simulink model "Bebop_controller_sim"  (R2018a)
settings: Solver=VariableStepAuto  StartTime=0.0  StopTime=25  RelTol=1e-3
values from neighbouring files (symbols this model uses):
  goal = [10 10]    [AnytimeRRT.m]    (also in Plot_sim.m = [rand()*5+20 rand()*-5]; RRTstardy.m = [9 9])
  I = [1 0 0 ... (first row only)    [Bebop_sim_init.m]
  mass = 2    [Bebop_sim_init.m]
  max_rot_Z = (90)*pi/180    (= 1.57079632679)    [Bebop_sim_init.m]
  max_theta_X = (40)*pi/180    (= 0.698131700798)    [Bebop_sim_init.m]
  max_theta_Y = (40)*pi/180    (= 0.698131700798)    [Bebop_sim_init.m]
  max_v_Z = 1.5    [Bebop_sim_init.m]
  start = [0 0]    [AnytimeRRT.m]    (also in Plot_sim.m; RRTstardy.m)
undefined symbols (not defined in the file or in its folder): data
libraries: simulink x6, aerolibactuator x2, shared6dof x1
settings Model: Creator=derek  LastModifiedBy=derek

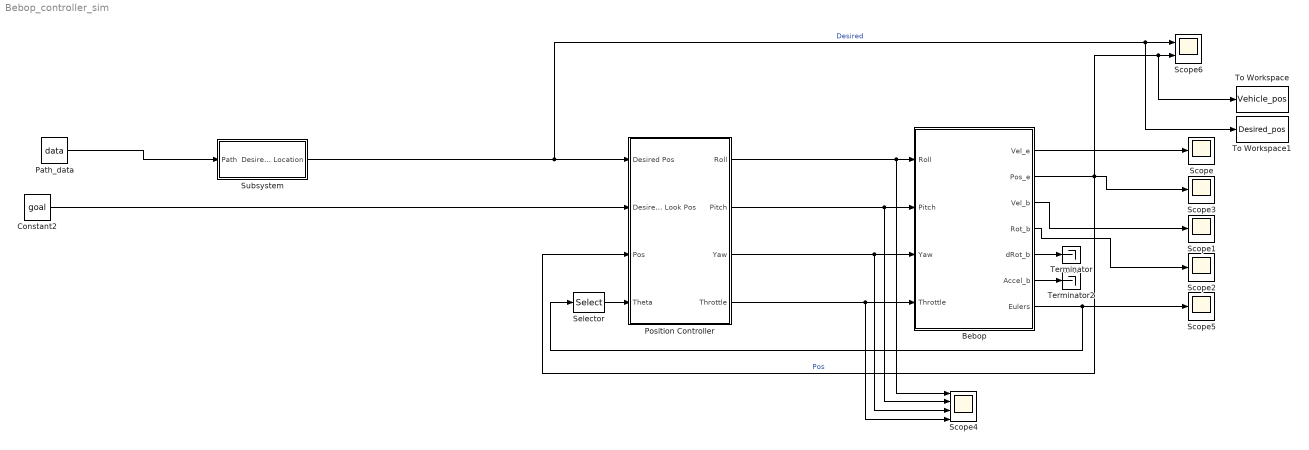
== system Bebop_controller_sim ==
  Bebop : Subsystem
  Constant2 : Constant  Value=goal
  Path_data : Constant  Value=data
  Position Controller : Subsystem
  Scope{,1..3,5} (5 alike) : Scope
  Scope4 : Scope  NumInputPorts=4
  Scope6 : Scope  NumInputPorts=2
  Selector : Selector  InputPortWidth=3  IndexOptions=Index vector (dialog)  Indices=[3]  OutputSizes=1
  Subsystem : Subsystem
  Terminator : Terminator
  Terminator2 : Terminator
  To Workspace : ToWorkspace  VariableName=Vehicle_pos  SaveFormat=Timeseries  SampleTime=-1
  To Workspace1 : ToWorkspace  VariableName=Desired_pos  SaveFormat=Timeseries  SampleTime=-1
  wires:
  Bebop/6(Accel_b) -> Terminator2/1
  Bebop/3(Vel_b) -> Scope1/1
  Position Controller/4(Throttle) -> Scope4/4, Bebop/4(Throttle)
  Bebop/5(dRot_b) -> Terminator/1
  Bebop/2(Pos_e) -> To Workspace/1, Scope6/2, Position Controller/3(Pos), Scope3/1  "Pos"
  Position Controller/3(Yaw) -> Scope4/3, Bebop/3(Yaw)
  Bebop/4(Rot_b) -> Scope2/1
  Position Controller/2(Pitch) -> Scope4/2, Bebop/2(Pitch)
  Bebop/1(Vel_e) -> Scope/1
  Position Controller/1(Roll) -> Scope4/1, Bebop/1(Roll)
  Subsystem/1(Desired Location) -> To Workspace1/1, Scope6/1, Position Controller/1(Desired Pos)  "Desired"
  Constant2/1 -> Position Controller/2(Desired Look Pos)
  Bebop/7(Eulers) -> Selector/1, Scope5/1
  Selector/1 -> Position Controller/4(Theta)
  Path_data/1 -> Subsystem/1(Path)

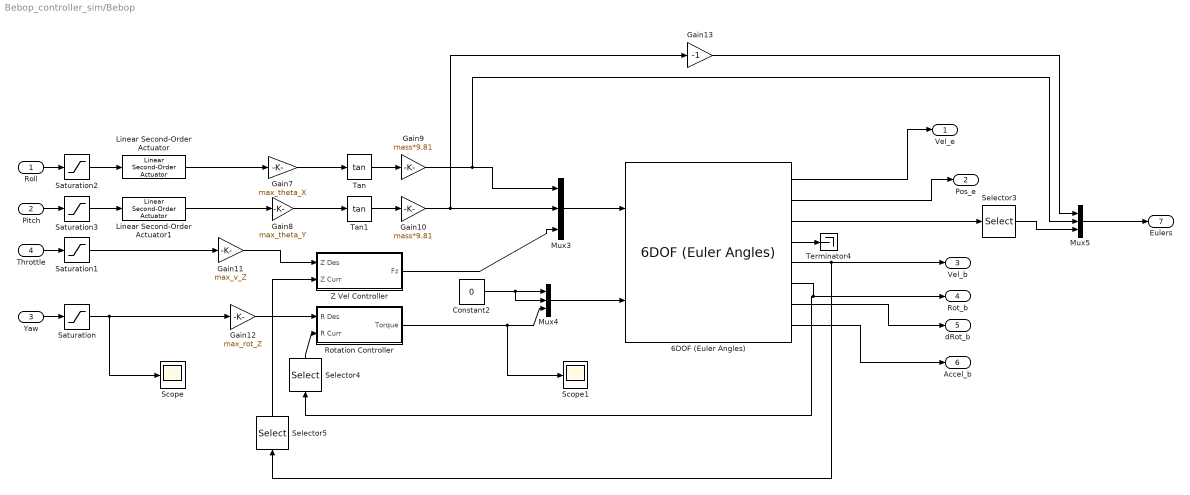
== system Bebop_controller_sim/Bebop ==
  Roll : Inport
  Pitch : Inport  Port=2
  Yaw : Inport  Port=3
  Throttle : Inport  Port=4
  6DOF (Euler Angles) : shared6dof/6DOF (Euler Angles)  units=Metric (MKS)  mtype=Fixed  rep=Euler Angles  xme_0=[start 3]  Vm_0=Initial_vel_b  eul_0=[0 0 0]  pm_0=[0 0 0]  mass_0=mass  mass_e=0.5  mass_f=2.0  inertia=I  inertia_e=eye(3)  inertia_f=2*eye(3)  k_quat=1.0  vre_flag=on  abi_flag=off  aMode=0
      settings: SourceProductBaseCode=AE
  Constant2 : Constant  Value=0
  Gain10 : Gain  Gain=mass*9.81
  Gain11 : Gain  Gain=max_v_Z
  Gain12 : Gain  Gain=max_rot_Z
  Gain13 : Gain  Gain=-1
  Gain7 : Gain  Gain=max_theta_X
  Gain8 : Gain  Gain=max_theta_Y
  Gain9 : Gain  Gain=mass*9.81
  Linear Second-Order Actuator : aerolibactuator/Linear Second-Order Actuator  wn_fin=20  z_fin=1  fin_act_0=0  fin_act_vel=0
      settings: SourceProductName=Aerospace Blockset  SourceProductBaseCode=AE
  Linear Second-Order Actuator1 : aerolibactuator/Linear Second-Order Actuator  wn_fin=20  z_fin=1  fin_act_0=0  fin_act_vel=0
      settings: SourceProductName=Aerospace Blockset  SourceProductBaseCode=AE
  Mux3 : Mux  Inputs=3
  Mux4 : Mux  Inputs=3
  Mux5 : Mux  Inputs=3
  Rotation Controller : Subsystem
  Saturation{,1..3} (4 alike) : Saturate  UpperLimit=1  LowerLimit=-1
  Scope : Scope
  Scope1 : Scope
  Selector3 : Selector  InputPortWidth=3  IndexOptions=Index vector (dialog)  Indices=3  OutputSizes=1
  Selector4 : Selector  InputPortWidth=3  IndexOptions=Index vector (dialog)  Indices=3  OutputSizes=1
  Selector5 : Selector  InputPortWidth=3  IndexOptions=Index vector (dialog)  Indices=3  OutputSizes=1
  Tan : Trigonometry  Operator=tan
  Tan1 : Trigonometry  Operator=tan
  Terminator4 : Terminator
  Z Vel Controller : Subsystem
  Vel_e : Outport
  Pos_e : Outport  Port=2
  Vel_b : Outport  Port=3
  Rot_b : Outport  Port=4
  dRot_b : Outport  Port=5
  Accel_b : Outport  Port=6
  Eulers : Outport  Port=7
  wires:
  Yaw/1 -> Saturation/1
  Gain12/1 -> Rotation Controller/1(R Des)
  Mux4/1 -> 6DOF (Euler Angles)/2
  Gain11/1 -> Z Vel Controller/1(Z Des)
  Throttle/1 -> Saturation1/1
  Pitch/1 -> Saturation3/1
  Gain10/1 -> Gain13/1, Mux3/2
  Tan/1 -> Gain9/1
  Constant2/1 -> Mux4/1, Mux4/2
  Gain8/1 -> Tan1/1
  Tan1/1 -> Gain10/1
  Rotation Controller/1(Torque) -> Scope1/1, Mux4/3
  Z Vel Controller/1(Fz) -> Mux3/3
  Gain7/1 -> Tan/1
  Roll/1 -> Saturation2/1
  6DOF (Euler Angles)/5 -> Selector5/1, Vel_b/1
  Mux3/1 -> 6DOF (Euler Angles)/1
  6DOF (Euler Angles)/6 -> Selector4/1, Rot_b/1
  6DOF (Euler Angles)/2 -> Pos_e/1
  6DOF (Euler Angles)/1 -> Vel_e/1
  6DOF (Euler Angles)/7 -> dRot_b/1
  6DOF (Euler Angles)/8 -> Accel_b/1
  6DOF (Euler Angles)/4 -> Terminator4/1
  Linear Second-Order Actuator/1 -> Gain7/1
  Linear Second-Order Actuator1/1 -> Gain8/1
  6DOF (Euler Angles)/3 -> Selector3/1
  Selector3/1 -> Mux5/3
  Gain13/1 -> Mux5/1
  Mux5/1 -> Eulers/1
  Gain9/1 -> Mux5/2, Mux3/1
  Selector4/1 -> Rotation Controller/2(R Curr)
  Selector5/1 -> Z Vel Controller/2(Z Curr)
  Saturation/1 -> Scope/1, Gain12/1
  Saturation1/1 -> Gain11/1
  Saturation2/1 -> Linear Second-Order Actuator/1
  Saturation3/1 -> Linear Second-Order Actuator1/1

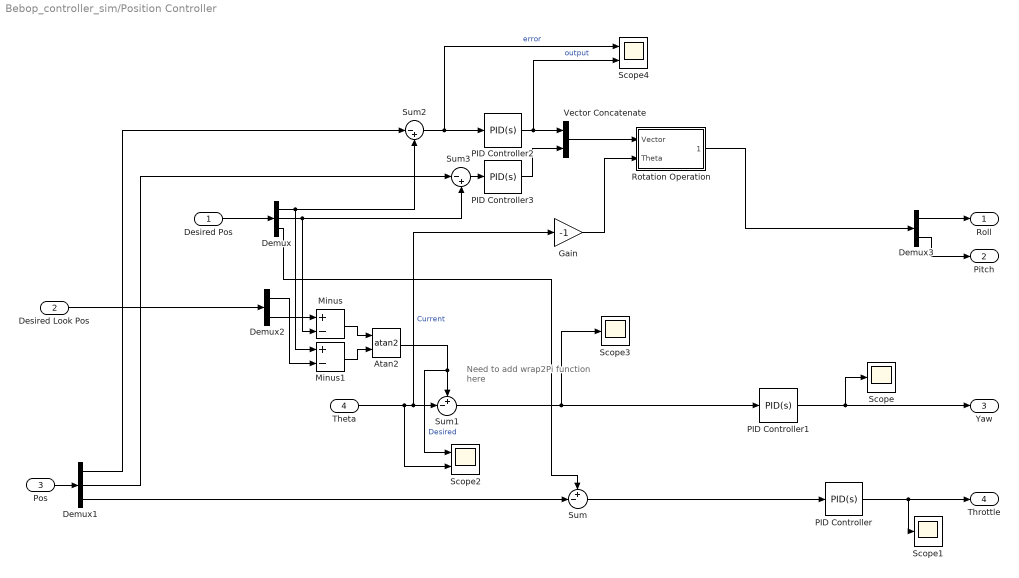
== system Bebop_controller_sim/Position Controller ==
  note: Need to add wrap2Pi function
      | here
  Desired Pos : Inport
  Desired Look Pos : Inport  Port=2
  Pos : Inport  Port=3
  Theta : Inport  Port=4
  Atan2 : Trigonometry  Operator=atan2
  Demux : Demux  Outputs=3
  Demux1 : Demux  Outputs=3
  Demux2 : Demux  Outputs=2
  Demux3 : Demux  Outputs=2
  Gain : Gain  Gain=-1
  Minus : Sum  Inputs=+-
  Minus1 : Sum  Inputs=+-
  PID Controller : simulink/Continuous/PID Controller  Controller=PID  TimeDomain=Continuous-time  SampleTime=-1  IntegratorMethod=Forward Euler  FilterMethod=Forward Euler  Form=Parallel  UseFilter=on  ControllerParametersSource=internal  P=3  I=0  D=.5  N=100  InitialConditionSource=internal  InitialConditionForIntegrator=0  InitialConditionForFilter=0  ExternalReset=none  LimitOutput=off  UpperSaturationLimit=inf  LowerSaturationLimit=-inf  LinearizeAsGain=on  AntiWindupMode=none  Kb=1  TrackingMode=off  Kt=1  PParamMin=[]  PParamMax=[]  IParamMin=[]  IParamMax=[]  DParamMin=[]  DParamMax=[]  NParamMin=[]  NParamMax=[]  KbParamMin=[]  KbParamMax=[]  KtParamMin=[]  KtParamMax=[]  POutMin=[]  POutMax=[]  IOutMin=[]  IOutMax=[]  DOutMin=[]  DOutMax=[]  NOutMin=[]  NOutMax=[]  KbOutMin=[]  KbOutMax=[]  KtOutMin=[]  KtOutMax=[]  IntegratorOutMin=[]  IntegratorOutMax=[]  FilterOutMin=[]  FilterOutMax=[]  SumOutMin=[]  SumOutMax=[]  SumI1OutMin=[]  SumI1OutMax=[]  SumI2OutMin=[]  SumI2OutMax=[]  SumI3OutMin=[]  SumI3OutMax=[]  SumDOutMin=[]  SumDOutMax=[]  SaturationOutMin=[]  SaturationOutMax=[]  IntegratorContinuousStateAttributes=''  IntegratorStateMustResolveToSignalObject=off  IntegratorRTWStateStorageClass=Auto  FilterContinuousStateAttributes=''  FilterStateMustResolveToSignalObject=off  FilterRTWStateStorageClass=Auto  DifferentiatorICPrevScaledInput=0  DifferentiatorOutMin=[]  DifferentiatorOutMax=[]  FilterDiffOutCoefMin=[]  FilterDiffOutCoefMax=[]  SumDenOutMin=[]  SumDenOutMax=[]  SumNumOutMin=[]  SumNumOutMax=[]  ReciprocalOutMin=[]  ReciprocalOutMax=[]  DivideOutMin=[]  DivideOutMax=[]  TunerSelectOption=Transfer Function Based (PID Tuner App)
  PID Controller1 : simulink/Continuous/PID Controller  Controller=PID  TimeDomain=Continuous-time  SampleTime=-1  IntegratorMethod=Forward Euler  FilterMethod=Forward Euler  Form=Parallel  UseFilter=on  ControllerParametersSource=internal  P=3  I=0  D=.5  N=100  InitialConditionSource=internal  InitialConditionForIntegrator=0  InitialConditionForFilter=0  ExternalReset=none  LimitOutput=off  UpperSaturationLimit=inf  LowerSaturationLimit=-inf  LinearizeAsGain=on  AntiWindupMode=none  Kb=1  TrackingMode=off  Kt=1  PParamMin=[]  PParamMax=[]  IParamMin=[]  IParamMax=[]  DParamMin=[]  DParamMax=[]  NParamMin=[]  NParamMax=[]  KbParamMin=[]  KbParamMax=[]  KtParamMin=[]  KtParamMax=[]  POutMin=[]  POutMax=[]  IOutMin=[]  IOutMax=[]  DOutMin=[]  DOutMax=[]  NOutMin=[]  NOutMax=[]  KbOutMin=[]  KbOutMax=[]  KtOutMin=[]  KtOutMax=[]  IntegratorOutMin=[]  IntegratorOutMax=[]  FilterOutMin=[]  FilterOutMax=[]  SumOutMin=[]  SumOutMax=[]  SumI1OutMin=[]  SumI1OutMax=[]  SumI2OutMin=[]  SumI2OutMax=[]  SumI3OutMin=[]  SumI3OutMax=[]  SumDOutMin=[]  SumDOutMax=[]  SaturationOutMin=[]  SaturationOutMax=[]  IntegratorContinuousStateAttributes=''  IntegratorStateMustResolveToSignalObject=off  IntegratorRTWStateStorageClass=Auto  FilterContinuousStateAttributes=''  FilterStateMustResolveToSignalObject=off  FilterRTWStateStorageClass=Auto  DifferentiatorICPrevScaledInput=0  DifferentiatorOutMin=[]  DifferentiatorOutMax=[]  FilterDiffOutCoefMin=[]  FilterDiffOutCoefMax=[]  SumDenOutMin=[]  SumDenOutMax=[]  SumNumOutMin=[]  SumNumOutMax=[]  ReciprocalOutMin=[]  ReciprocalOutMax=[]  DivideOutMin=[]  DivideOutMax=[]  TunerSelectOption=Transfer Function Based (PID Tuner App)
  PID Controller2 : simulink/Continuous/PID Controller  Controller=PID  TimeDomain=Continuous-time  SampleTime=-1  IntegratorMethod=Forward Euler  FilterMethod=Forward Euler  Form=Parallel  UseFilter=on  ControllerParametersSource=internal  P=.1  I=0  D=.12  N=100  InitialConditionSource=internal  InitialConditionForIntegrator=0  InitialConditionForFilter=0  ExternalReset=none  LimitOutput=off  UpperSaturationLimit=inf  LowerSaturationLimit=-inf  LinearizeAsGain=on  AntiWindupMode=none  Kb=1  TrackingMode=off  Kt=1  PParamMin=[]  PParamMax=[]  IParamMin=[]  IParamMax=[]  DParamMin=[]  DParamMax=[]  NParamMin=[]  NParamMax=[]  KbParamMin=[]  KbParamMax=[]  KtParamMin=[]  KtParamMax=[]  POutMin=[]  POutMax=[]  IOutMin=[]  IOutMax=[]  DOutMin=[]  DOutMax=[]  NOutMin=[]  NOutMax=[]  KbOutMin=[]  KbOutMax=[]  KtOutMin=[]  KtOutMax=[]  IntegratorOutMin=[]  IntegratorOutMax=[]  FilterOutMin=[]  FilterOutMax=[]  SumOutMin=[]  SumOutMax=[]  SumI1OutMin=[]  SumI1OutMax=[]  SumI2OutMin=[]  SumI2OutMax=[]  SumI3OutMin=[]  SumI3OutMax=[]  SumDOutMin=[]  SumDOutMax=[]  SaturationOutMin=[]  SaturationOutMax=[]  IntegratorContinuousStateAttributes=''  IntegratorStateMustResolveToSignalObject=off  IntegratorRTWStateStorageClass=Auto  FilterContinuousStateAttributes=''  FilterStateMustResolveToSignalObject=off  FilterRTWStateStorageClass=Auto  DifferentiatorICPrevScaledInput=0  DifferentiatorOutMin=[]  DifferentiatorOutMax=[]  FilterDiffOutCoefMin=[]  FilterDiffOutCoefMax=[]  SumDenOutMin=[]  SumDenOutMax=[]  SumNumOutMin=[]  SumNumOutMax=[]  ReciprocalOutMin=[]  ReciprocalOutMax=[]  DivideOutMin=[]  DivideOutMax=[]  TunerSelectOption=Transfer Function Based (PID Tuner App)
  PID Controller3 : simulink/Continuous/PID Controller  Controller=PID  TimeDomain=Continuous-time  SampleTime=-1  IntegratorMethod=Forward Euler  FilterMethod=Forward Euler  Form=Parallel  UseFilter=on  ControllerParametersSource=internal  P=.1  I=0  D=.12  N=100  InitialConditionSource=internal  InitialConditionForIntegrator=0  InitialConditionForFilter=0  ExternalReset=none  LimitOutput=off  UpperSaturationLimit=inf  LowerSaturationLimit=-inf  LinearizeAsGain=on  AntiWindupMode=none  Kb=1  TrackingMode=off  Kt=1  PParamMin=[]  PParamMax=[]  IParamMin=[]  IParamMax=[]  DParamMin=[]  DParamMax=[]  NParamMin=[]  NParamMax=[]  KbParamMin=[]  KbParamMax=[]  KtParamMin=[]  KtParamMax=[]  POutMin=[]  POutMax=[]  IOutMin=[]  IOutMax=[]  DOutMin=[]  DOutMax=[]  NOutMin=[]  NOutMax=[]  KbOutMin=[]  KbOutMax=[]  KtOutMin=[]  KtOutMax=[]  IntegratorOutMin=[]  IntegratorOutMax=[]  FilterOutMin=[]  FilterOutMax=[]  SumOutMin=[]  SumOutMax=[]  SumI1OutMin=[]  SumI1OutMax=[]  SumI2OutMin=[]  SumI2OutMax=[]  SumI3OutMin=[]  SumI3OutMax=[]  SumDOutMin=[]  SumDOutMax=[]  SaturationOutMin=[]  SaturationOutMax=[]  IntegratorContinuousStateAttributes=''  IntegratorStateMustResolveToSignalObject=off  IntegratorRTWStateStorageClass=Auto  FilterContinuousStateAttributes=''  FilterStateMustResolveToSignalObject=off  FilterRTWStateStorageClass=Auto  DifferentiatorICPrevScaledInput=0  DifferentiatorOutMin=[]  DifferentiatorOutMax=[]  FilterDiffOutCoefMin=[]  FilterDiffOutCoefMax=[]  SumDenOutMin=[]  SumDenOutMax=[]  SumNumOutMin=[]  SumNumOutMax=[]  ReciprocalOutMin=[]  ReciprocalOutMax=[]  DivideOutMin=[]  DivideOutMax=[]  TunerSelectOption=Transfer Function Based (PID Tuner App)
  Rotation Operation : Subsystem
  Scope : Scope
  Scope1 : Scope
  Scope2 : Scope  NumInputPorts=2
  Scope3 : Scope
  Scope4 : Scope  NumInputPorts=2
  Sum : Sum  Inputs=+-|
  Sum1 : Sum  Inputs=+-|
  Sum2 : Sum  Inputs=|-+
  Sum3 : Sum  Inputs=|-+
  Vector Concatenate : Concatenate
  Roll : Outport
  Pitch : Outport  Port=2
  Yaw : Outport  Port=3
  Throttle : Outport  Port=4
  wires:
  Desired Pos/1 -> Demux/1
  PID Controller/1 -> Scope1/1, Throttle/1
  Demux/3 -> Sum/1
  Pos/1 -> Demux1/1
  Demux1/3 -> Sum/2
  Sum/1 -> PID Controller/1
  Desired Look Pos/1 -> Demux2/1
  Demux/2 -> Sum3/2, Minus/1
  Demux2/2 -> Minus/2
  Minus/1 -> Atan2/1
  Demux2/1 -> Minus1/2
  Demux/1 -> Sum2/2, Minus1/1
  Minus1/1 -> Atan2/2
  Atan2/1 -> Scope2/1, Sum1/1  "Desired"
  Theta/1 -> Gain/1, Sum1/2, Scope2/2  "Current"
  Sum1/1 -> Scope3/1, PID Controller1/1
  PID Controller1/1 -> Scope/1, Yaw/1
  Demux1/1 -> Sum2/1
  Demux1/2 -> Sum3/1
  Sum2/1 -> Scope4/1, PID Controller2/1  "error"
  Sum3/1 -> PID Controller3/1
  PID Controller2/1 -> Scope4/2, Vector Concatenate/1  "output"
  PID Controller3/1 -> Vector Concatenate/2
  Vector Concatenate/1 -> Rotation Operation/1(Vector)
  Rotation Operation/1(Vec New) -> Demux3/1
  Demux3/1 -> Roll/1
  Demux3/2 -> Pitch/1
  Gain/1 -> Rotation Operation/2(Theta)

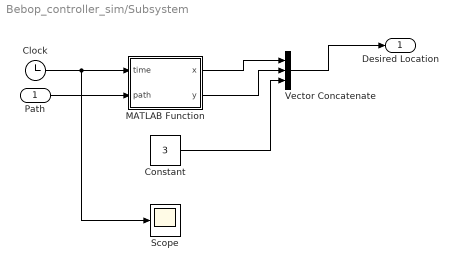
== system Bebop_controller_sim/Subsystem ==
  Path : Inport
  Clock : Clock
  Constant : Constant  Value=3
  MATLAB Function : MATLAB Function  TreatAsAtomicUnit=on
  Scope : Scope
  Vector Concatenate : Concatenate  NumInputs=3
  Desired Location : Outport
  wires:
  Constant/1 -> Vector Concatenate/3
  Vector Concatenate/1 -> Desired Location/1
  Path/1 -> MATLAB Function/2(path)
  MATLAB Function/1(x) -> Vector Concatenate/1
  MATLAB Function/2(y) -> Vector Concatenate/2
  Clock/1 -> Scope/1, MATLAB Function/1(time)

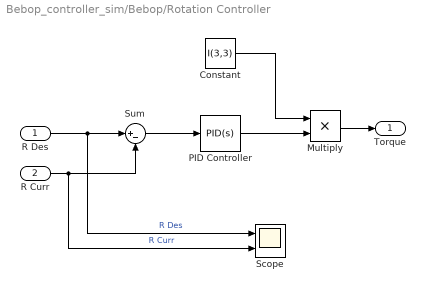
== system Bebop_controller_sim/Bebop/Rotation Controller ==
  R Des : Inport
  R Curr : Inport  Port=2
  Constant : Constant  Value=I(3,3)
  Multiply : Product
  PID Controller : simulink/Continuous/PID Controller  Controller=PID  TimeDomain=Continuous-time  SampleTime=-1  IntegratorMethod=Forward Euler  FilterMethod=Forward Euler  Form=Parallel  UseFilter=on  ControllerParametersSource=internal  P=10  I=.3  D=.1  N=100  InitialConditionSource=internal  InitialConditionForIntegrator=0  InitialConditionForFilter=0  ExternalReset=none  LimitOutput=off  UpperSaturationLimit=inf  LowerSaturationLimit=-inf  LinearizeAsGain=on  AntiWindupMode=none  Kb=1  TrackingMode=off  Kt=1  PParamMin=[]  PParamMax=[]  IParamMin=[]  IParamMax=[]  DParamMin=[]  DParamMax=[]  NParamMin=[]  NParamMax=[]  KbParamMin=[]  KbParamMax=[]  KtParamMin=[]  KtParamMax=[]  POutMin=[]  POutMax=[]  IOutMin=[]  IOutMax=[]  DOutMin=[]  DOutMax=[]  NOutMin=[]  NOutMax=[]  KbOutMin=[]  KbOutMax=[]  KtOutMin=[]  KtOutMax=[]  IntegratorOutMin=[]  IntegratorOutMax=[]  FilterOutMin=[]  FilterOutMax=[]  SumOutMin=[]  SumOutMax=[]  SumI1OutMin=[]  SumI1OutMax=[]  SumI2OutMin=[]  SumI2OutMax=[]  SumI3OutMin=[]  SumI3OutMax=[]  SumDOutMin=[]  SumDOutMax=[]  SaturationOutMin=[]  SaturationOutMax=[]  IntegratorContinuousStateAttributes=''  IntegratorStateMustResolveToSignalObject=off  IntegratorRTWStateStorageClass=Auto  FilterContinuousStateAttributes=''  FilterStateMustResolveToSignalObject=off  FilterRTWStateStorageClass=Auto  DifferentiatorICPrevScaledInput=0  DifferentiatorOutMin=[]  DifferentiatorOutMax=[]  FilterDiffOutCoefMin=[]  FilterDiffOutCoefMax=[]  SumDenOutMin=[]  SumDenOutMax=[]  SumNumOutMin=[]  SumNumOutMax=[]  ReciprocalOutMin=[]  ReciprocalOutMax=[]  DivideOutMin=[]  DivideOutMax=[]  TunerSelectOption=Transfer Function Based (PID Tuner App)
  Scope : Scope  NumInputPorts=2
  Sum : Sum  Inputs=|+-
  Torque : Outport
  wires:
  R Des/1 -> Scope/1, Sum/1  "R Des"
  PID Controller/1 -> Multiply/2
  Sum/1 -> PID Controller/1
  Multiply/1 -> Torque/1
  R Curr/1 -> Scope/2, Sum/2  "R Curr"
  Constant/1 -> Multiply/1

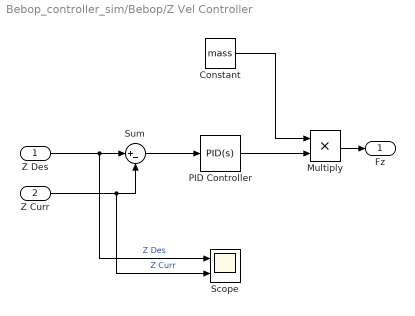
== system Bebop_controller_sim/Bebop/Z Vel Controller ==
  Z Des : Inport
  Z Curr : Inport  Port=2
  Constant : Constant  Value=mass
  Multiply : Product
  PID Controller : simulink/Continuous/PID Controller  Controller=PID  TimeDomain=Continuous-time  SampleTime=-1  IntegratorMethod=Forward Euler  FilterMethod=Forward Euler  Form=Parallel  UseFilter=on  ControllerParametersSource=internal  P=5  I=.15  D=.1  N=100  InitialConditionSource=internal  InitialConditionForIntegrator=0  InitialConditionForFilter=0  ExternalReset=none  LimitOutput=off  UpperSaturationLimit=inf  LowerSaturationLimit=-inf  LinearizeAsGain=on  AntiWindupMode=none  Kb=1  TrackingMode=off  Kt=1  PParamMin=[]  PParamMax=[]  IParamMin=[]  IParamMax=[]  DParamMin=[]  DParamMax=[]  NParamMin=[]  NParamMax=[]  KbParamMin=[]  KbParamMax=[]  KtParamMin=[]  KtParamMax=[]  POutMin=[]  POutMax=[]  IOutMin=[]  IOutMax=[]  DOutMin=[]  DOutMax=[]  NOutMin=[]  NOutMax=[]  KbOutMin=[]  KbOutMax=[]  KtOutMin=[]  KtOutMax=[]  IntegratorOutMin=[]  IntegratorOutMax=[]  FilterOutMin=[]  FilterOutMax=[]  SumOutMin=[]  SumOutMax=[]  SumI1OutMin=[]  SumI1OutMax=[]  SumI2OutMin=[]  SumI2OutMax=[]  SumI3OutMin=[]  SumI3OutMax=[]  SumDOutMin=[]  SumDOutMax=[]  SaturationOutMin=[]  SaturationOutMax=[]  IntegratorContinuousStateAttributes=''  IntegratorStateMustResolveToSignalObject=off  IntegratorRTWStateStorageClass=Auto  FilterContinuousStateAttributes=''  FilterStateMustResolveToSignalObject=off  FilterRTWStateStorageClass=Auto  DifferentiatorICPrevScaledInput=0  DifferentiatorOutMin=[]  DifferentiatorOutMax=[]  FilterDiffOutCoefMin=[]  FilterDiffOutCoefMax=[]  SumDenOutMin=[]  SumDenOutMax=[]  SumNumOutMin=[]  SumNumOutMax=[]  ReciprocalOutMin=[]  ReciprocalOutMax=[]  DivideOutMin=[]  DivideOutMax=[]  TunerSelectOption=Transfer Function Based (PID Tuner App)
  Scope : Scope  NumInputPorts=2
  Sum : Sum  Inputs=|+-
  Fz : Outport
  wires:
  Z Des/1 -> Scope/1, Sum/1  "Z Des"
  Z Curr/1 -> Scope/2, Sum/2  "Z Curr"
  Sum/1 -> PID Controller/1
  Multiply/1 -> Fz/1
  PID Controller/1 -> Multiply/2
  Constant/1 -> Multiply/1

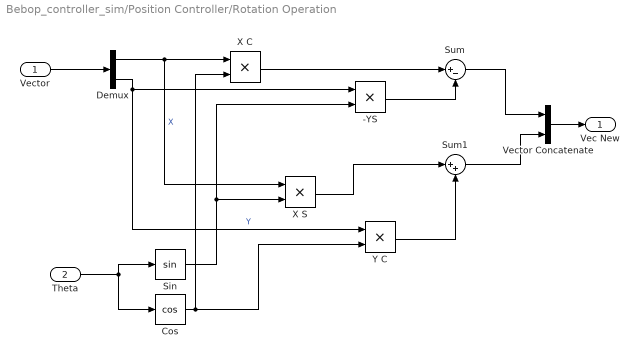
== system Bebop_controller_sim/Position Controller/Rotation Operation ==
  Vector : Inport
  Theta : Inport  Port=2
  -YS : Product
  Cos : Trigonometry  Operator=cos
  Demux : Demux  Outputs=2
  Sin : Trigonometry
  Sum : Sum  Inputs=|+-
  Sum1 : Sum  Inputs=|++
  Vector Concatenate : Concatenate
  X C : Product
  X S : Product
  Y C : Product
  Vec New : Outport
  wires:
  Vector/1 -> Demux/1
  Theta/1 -> Sin/1, Cos/1
  Demux/1 -> X S/1, X C/1  "X"
  Demux/2 -> Y C/1, -YS/1  "Y"
  Vector Concatenate/1 -> Vec New/1
  Sum/1 -> Vector Concatenate/1
  Sum1/1 -> Vector Concatenate/2
  X C/1 -> Sum/1
  -YS/1 -> Sum/2
  X S/1 -> Sum1/1
  Sin/1 -> X S/2, -YS/2
  Cos/1 -> Y C/2, X C/2
  Y C/1 -> Sum1/2

== matlab function Bebop_controller_sim/Subsystem/MATLAB Function ==
  data: time input; path input; x output; y output
function [x,y]= fcn(time,path)
    indx = size(path,1);
    for k = 2:size(path,1)
        if time < path(k,1)
            indx = k-1;
            break
        end
    end
    x = path(indx,2);
    y = path(indx,3);
end
